simulink model "TestCode"  (R2015a)
settings: Solver=ode45  StartTime=0.0  StopTime=10.0  RelTol=1e-3
settings Model: Creator=admin  LastModifiedBy=admin

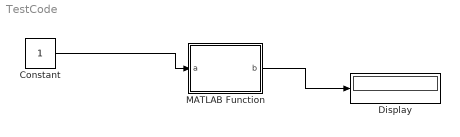
== system TestCode ==
  Constant : Constant
  Display : Display
  MATLAB Function : MATLAB Function  TreatAsAtomicUnit=on
  wires:
  Constant/1 -> MATLAB Function/1(a)
  MATLAB Function/1(b) -> Display/1

== matlab function TestCode/MATLAB Function ==
  data: a input; b output
function b = fcn(a)
%#codegen
%mat= zeros(3,3);
%for i=1:3
 %   for j=1:3
  %      mat(i,j)=a+i+j;
   % end
%end

b=a+1;

end
